simulink model "dop1"  (R2018b)
settings: Solver=ode45  StartTime=0.0  StopTime=15  RelTol=1e-3  EnableMultiTasking=on
libraries: simulink x2
settings Model: Creator=bukova.2018  LastModifiedBy=Kirill
settings DataIOCC: LimitDataPoints=on  SaveFormat=Array
settings OptimizationCC: LifeSpan=inf
settings DebuggingCC: SolverPrmCheckMsg=warning  LibraryContextMissingDiagnostic=none  SFUnexpectedBacktrackingDiag=warning  SFNoUnconditionalDefaultTransitionDiag=warning  SFExecutionAtInitializationDiag=none
settings HardwareCC: ProdBitPerPointer=32  ProdBitPerSizeT=32  ProdBitPerPtrDiffT=32  ProdLargestAtomicFloat=None  ProdIntDivRoundTo=Undefined  ProdEndianess=Unspecified  ProdWordSize=32  ProdHWDeviceType=32-bit Generic
settings ModelReferenceCC: PropagateSignalLabelsOutOfModel=off
settings SFSimCC: SimUseLocalCustomCode=off
settings RTWCC: RTWUseLocalCustomCode=off
settings CodeAppCC: StateflowObjectComments=on
settings GRTTargetCC: TargetLangStandard=C89/C90 (ANSI)  GeneratePreprocessorConditionals=Disable all
settings ConfigComp: CovMetricSettings=dw  CovHtmlReporting=on  CovSaveCumulativeToWorkspaceVar=on  CovSaveSingleToWorkspaceVar=on  CovExternalEMLEnable=off  CovSFcnEnable=off

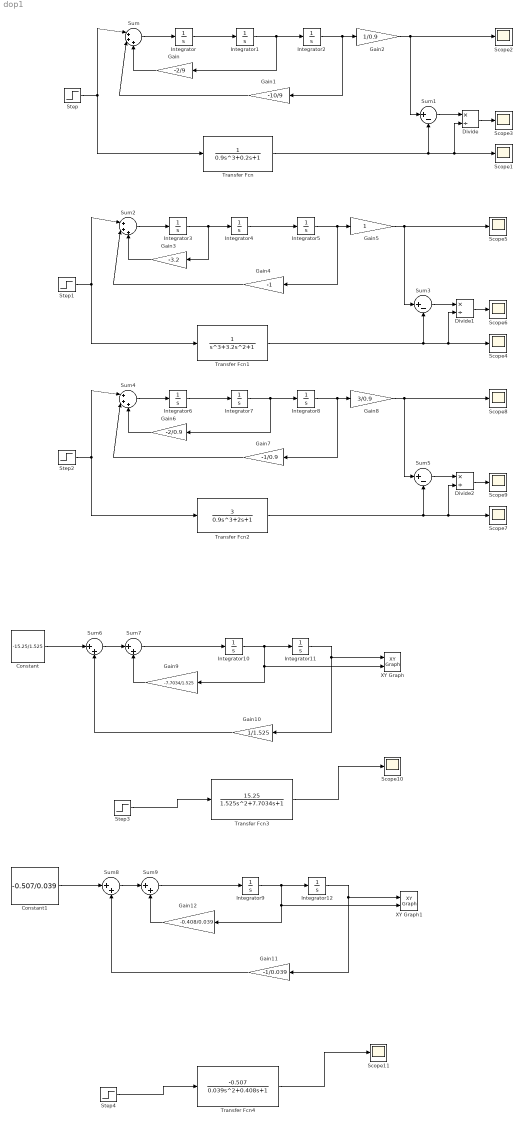
== system dop1 ==
  Constant : Constant  Value=-15.25/1.525
  Constant1 : Constant  Value=-0.507/0.039
  Divide : Product  Inputs=*/
  Divide1 : Product  Inputs=*/
  Divide2 : Product  Inputs=*/
  Gain : Gain  Gain=-2/9
  Gain1 : Gain  Gain=-10/9
  Gain10 : Gain  Gain=1/1.525
  Gain11 : Gain  Gain=-1/0.039
  Gain12 : Gain  Gain=-0.408/0.039
  Gain2 : Gain  Gain=1/0.9
  Gain3 : Gain  Gain=-3.2
  Gain4 : Gain  Gain=-1
  Gain5 : Gain
  Gain6 : Gain  Gain=-2/0.9
  Gain7 : Gain  Gain=-1/0.9
  Gain8 : Gain  Gain=3/0.9
  Gain9 : Gain  Gain=-7.7034/1.525
  Integrator{,1..8} (9 alike) : Integrator
  Integrator10 : Integrator  InitialCondition=1
  Integrator11 : Integrator  InitialCondition=-1
  Integrator12 : Integrator  InitialCondition=10000
  Integrator9 : Integrator  InitialCondition=-200
  Scope{1..11} (11 alike) : Scope
  Step : Step  SampleTime=0
  Step1 : Step  SampleTime=0
  Step2 : Step  SampleTime=0
  Step3 : Step  Time=0  SampleTime=0
  Step4 : Step  Time=0  SampleTime=0
  Sum : Sum  Inputs=|+++
  Sum1 : Sum  Inputs=|+-
  Sum2 : Sum  Inputs=|+++
  Sum3 : Sum  Inputs=|+-
  Sum4 : Sum  Inputs=|+++
  Sum5 : Sum  Inputs=|+-
  Sum{6..9} (4 alike) : Sum  Inputs=|++
  Transfer Fcn : TransferFcn  Denominator=[0.9 0 0.2 1]
  Transfer Fcn1 : TransferFcn  Denominator=[1 3.2 0 1]
  Transfer Fcn2 : TransferFcn  Numerator=[3]  Denominator=[0.9 0 2 1]
  Transfer Fcn3 : TransferFcn  Numerator=[15.25]  Denominator=[1.525 7.7034 1]
  Transfer Fcn4 : TransferFcn  Numerator=[-0.507]  Denominator=[0.039 0.408 1]
  XY Graph : simulink/Sinks/XY Graph  xmin=-1000  xmax=1000  ymin=-1000  ymax=1000  st=-1
  XY Graph1 : simulink/Sinks/XY Graph  xmin=-1000  xmax=1000  ymin=-1000  ymax=1000  st=-1
  wires:
  Integrator1/1 -> Gain/1, Integrator2/1
  Gain1/1 -> Sum/2
  Gain/1 -> Sum/3
  Integrator/1 -> Integrator1/1
  Sum/1 -> Integrator/1
  Divide/1 -> Scope3/1
  Transfer Fcn/1 -> Scope1/1, Divide/2, Sum1/2
  Step/1 -> Sum/1, Transfer Fcn/1
  Sum1/1 -> Divide/1
  Integrator2/1 -> Gain2/1, Gain1/1
  Gain2/1 -> Scope2/1, Sum1/1
  Gain4/1 -> Sum2/2
  Integrator3/1 -> Gain3/1, Integrator4/1
  Gain5/1 -> Scope5/1, Sum3/1
  Sum3/1 -> Divide1/1
  Sum2/1 -> Integrator3/1
  Integrator4/1 -> Integrator5/1
  Step1/1 -> Sum2/1, Transfer Fcn1/1
  Divide1/1 -> Scope6/1
  Integrator5/1 -> Gain5/1, Gain4/1
  Transfer Fcn1/1 -> Scope4/1, Divide1/2, Sum3/2
  Gain3/1 -> Sum2/3
  Sum5/1 -> Divide2/1
  Integrator6/1 -> Integrator7/1
  Gain7/1 -> Sum4/2
  Gain6/1 -> Sum4/3
  Transfer Fcn2/1 -> Scope7/1, Divide2/2, Sum5/2
  Gain8/1 -> Scope8/1, Sum5/1
  Integrator8/1 -> Gain8/1, Gain7/1
  Step2/1 -> Sum4/1, Transfer Fcn2/1
  Divide2/1 -> Scope9/1
  Sum4/1 -> Integrator6/1
  Integrator7/1 -> Gain6/1, Integrator8/1
  Integrator11/1 -> Gain10/1, XY Graph/1
  Sum7/1 -> Integrator10/1
  Integrator10/1 -> Gain9/1, XY Graph/2, Integrator11/1
  Sum6/1 -> Sum7/1
  Constant/1 -> Sum6/1
  Gain10/1 -> Sum6/2
  Gain9/1 -> Sum7/2
  Step3/1 -> Transfer Fcn3/1
  Transfer Fcn3/1 -> Scope10/1
  Constant1/1 -> Sum8/1
  Sum9/1 -> Integrator9/1
  Step4/1 -> Transfer Fcn4/1
  Gain11/1 -> Sum8/2
  Gain12/1 -> Sum9/2
  Integrator12/1 -> Gain11/1, XY Graph1/1
  Integrator9/1 -> Gain12/1, XY Graph1/2, Integrator12/1
  Sum8/1 -> Sum9/1
  Transfer Fcn4/1 -> Scope11/1
